simulink model "CryoDetFP"  (R2015b)
settings: Solver=ode45  SolverMode=SingleTasking  StartTime=0.0  StopTime=10e-5  MaxStep=1e-9  RelTol=1e-3
values from neighbouring files (symbols this model uses):
  Fclk = Fadc/2    (= 185000000)    [setupCryoFPGA.m]    (also in setupCryoNew.m)
  freqBusAddrBits = 4    [setupCryoNew.m]
  noise = ifft(exp(2i*pi*rand(1, noiseLen)) .* fft(fir1(noiseLen-1, noiseBW/Fclk*noiseSteps)))    [setupCryoFPGA.m]    (also in setupCryoNew.m = exp(2i*pi*rand(1, noiseLen)))
  noiseLen = 128    [setupCryoFPGA.m]    (also in setupCryoNew.m)
  noiseSteps = 32    [setupCryoFPGA.m]    (also in setupCryoNew.m)
  notch = tf( [1 a*wNotch/Q wNotch^2], [1 wNotch/Q wNotch^2])    [setupCryoNew.m]
  notch2 = tf( [1 a*wNotch/Q wNotch^2], [1 wNotch/Q wNotch^2])    [setupCryoNew.m]
  Tclk = 1/Fclk    (= 5.40540540541e-09)    [setupCryoFPGA.m]    (also in setupCryoNew.m)
undefined symbols (not defined in the file or in its folder): AXI4, Lite, notch3, notch4, xlipgetpartsetting
libraries: xbsIndex_r4 x1085
(part 1 of 8)
settings Model: Creator=ssmith  LastModifiedBy=ssmith
settings DataIOCC: SaveFormat=Array
settings OptimizationCC: BlockReduction=off  BooleanDataType=off
settings DebuggingCC: SaveWithParameterizedLinksMsg=none  UnderspecifiedInitializationDetection=Classic  MergeDetectMultiDrivingBlocksExec=none  SignalResolutionControl=TryResolveAllWithWarning
settings HardwareCC: ProdBitPerPointer=32  ProdLargestAtomicFloat=None  ProdIntDivRoundTo=Undefined  ProdEndianess=Unspecified  ProdWordSize=32  ProdHWDeviceType=32-bit Generic  TargetUnknown=on
settings GRTTargetCC: GeneratePreprocessorConditionals=Disable all
settings ConfigComp: CovModelRefEnable=Off  CovSFcnEnable=off

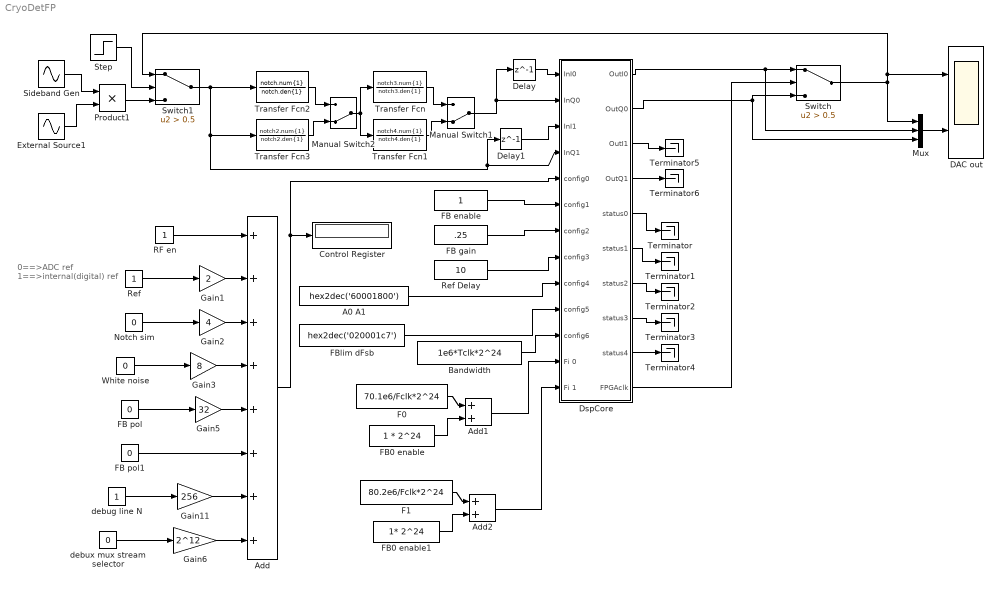
== system CryoDetFP ==
  note: 0==>ADC ref
      | 1==>internal(digital) ref
  A0 A1 : Constant  Value=hex2dec('60001800')  SampleTime=Tclk
  Add : Sum  Inputs=++++++++
  Add1 : Sum
  Add2 : Sum
  Bandwidth : Constant  Value=1e6*Tclk*2^24  SampleTime=Tclk
  Control Register : Display
      settings: Format=hex (Stored Integer)  Decimation=1000
  DAC out : Scope  NumInputPorts=2
  Delay : Delay  DelayLength=1  SampleTime=Tclk/2
  Delay1 : Delay  DelayLength=1  SampleTime=Tclk/2
  DspCore : Subsystem
  External Source1 : Sin  Amplitude=.8  Frequency=2*pi*70.1e6  SampleTime=0
  F0 : Constant  Value=70.1e6/Fclk*2^24  SampleTime=Tclk
  F1 : Constant  Value=80.2e6/Fclk*2^24  SampleTime=Tclk
  FB enable : Constant  SampleTime=Tclk
  FB gain : Constant  Value=.25  SampleTime=Tclk
  FB pol : Constant  Value=0  SampleTime=Tclk
  FB pol1 : Constant  Value=0  SampleTime=Tclk
  FB0 enable : Constant  Value=1 * 2^24  SampleTime=Tclk
  FB0 enable1 : Constant  Value=1* 2^24  SampleTime=Tclk
  FBlim dFsb : Constant  Value=hex2dec('020001c7')  SampleTime=Tclk
  Gain1 : Gain  Gain=2
  Gain11 : Gain  Gain=256
  Gain2 : Gain  Gain=4
  Gain3 : Gain  Gain=8
  Gain5 : Gain  Gain=32
  Gain6 : Gain  Gain=2^12
  Manual Switch1 : ManualSwitch  CurrentSetting=0
  Manual Switch2 : ManualSwitch  CurrentSetting=0
  Mux : Mux  Inputs=3
  Notch sim : Constant  Value=0  SampleTime=Tclk
  Product1 : Product
  RF en : Constant  SampleTime=Tclk
  Ref : Constant  SampleTime=Tclk
  Ref Delay : Constant  Value=10  SampleTime=Tclk
  Sideband Gen : Sin  Amplitude=0.24  Bias=0.75  Frequency=2*pi*1.284e6  SampleTime=0
  Step : Step  Time=1e-5  SampleTime=0
  Switch : Switch  Criteria=u2 > Threshold  Threshold=0.5
  Switch1 : Switch  Criteria=u2 > Threshold  Threshold=0.5
  Terminator{,1..6} (7 alike) : Terminator
  Transfer Fcn : TransferFcn  Numerator=notch3.num{1}  Denominator=notch3.den{1}
  Transfer Fcn1 : TransferFcn  Numerator=notch4.num{1}  Denominator=notch4.den{1}
  Transfer Fcn2 : TransferFcn  Numerator=notch.num{1}  Denominator=notch.den{1}
  Transfer Fcn3 : TransferFcn  Numerator=notch2.num{1}  Denominator=notch2.den{1}
  White noise : Constant  Value=0  SampleTime=Tclk
  debug line N : Constant  SampleTime=Tclk
  debux mux stream selector : Constant  Value=0  SampleTime=Tclk
  wires:
  Add/1 -> DspCore/5(config0), Control Register/1
  FB enable/1 -> DspCore/6(config1)
  DspCore/5(status0) -> Terminator/1
  DspCore/6(status1) -> Terminator1/1
  DspCore/7(status2) -> Terminator2/1
  DspCore/8(status3) -> Terminator3/1
  DspCore/9(status4) -> Terminator4/1
  Sideband Gen/1 -> Product1/1
  DspCore/10(FPGAclk) -> Switch/2
  DspCore/2(OutQ0) -> Switch/3, Mux/3
  Switch/1 -> DAC out/1, Switch1/1, Mux/1
  DspCore/1(OutI0) -> Switch/1, Mux/2
  Product1/1 -> Switch1/3
  Step/1 -> Switch1/2
  Manual Switch1/1 -> Delay/1, DspCore/2(InQ0)
  External Source1/1 -> Product1/2
  Transfer Fcn1/1 -> Manual Switch1/2
  Transfer Fcn/1 -> Manual Switch1/1
  RF en/1 -> Add/1
  Ref/1 -> Gain1/1
  Notch sim/1 -> Gain2/1
  White noise/1 -> Gain3/1
  FB pol/1 -> Gain5/1
  debux mux stream selector/1 -> Gain6/1
  Gain1/1 -> Add/2
  Gain2/1 -> Add/3
  Gain3/1 -> Add/4
  debug line N/1 -> Gain11/1
  Mux/1 -> DAC out/2
  Delay/1 -> DspCore/1(InI0)
  Delay1/1 -> DspCore/3(InI1)
  Gain11/1 -> Add/7
  Gain6/1 -> Add/8
  Gain5/1 -> Add/5
  FB gain/1 -> DspCore/7(config2)
  Ref Delay/1 -> DspCore/8(config3)
  A0 A1/1 -> DspCore/9("config4 ")
  FBlim dFsb/1 -> DspCore/10(config5)
  Bandwidth/1 -> DspCore/11(config6)
  FB pol1/1 -> Add/6
  FB0 enable/1 -> Add1/2
  F0/1 -> Add1/1
  Add1/1 -> DspCore/12(Fi 0)
  DspCore/3(OutI1) -> Terminator5/1
  DspCore/4(OutQ1) -> Terminator6/1
  Transfer Fcn3/1 -> Manual Switch2/2
  Transfer Fcn2/1 -> Manual Switch2/1
  Switch1/1 -> Transfer Fcn2/1, Transfer Fcn3/1, Delay1/1, DspCore/4(InQ1)
  Manual Switch2/1 -> Transfer Fcn/1, Transfer Fcn1/1
  FB0 enable1/1 -> Add2/2
  F1/1 -> Add2/1
  Add2/1 -> DspCore/13(Fi 1)

== system CryoDetFP/DspCore ==
  note: create an edge to synchronize external DAC interleaver simulation in Simulink
  note: DAC outputs
      | 16 bits
  note: ADC Inputs
      | 16 bits
      | 370 MSPS
  note: FPGA reset
  InI0 : Inport
  InQ0 : Inport  Port=2
  InI1 : Inport  Port=3
  InQ1 : Inport  Port=4
  config0 : Inport  Port=5
  config1 : Inport  Port=6
  config2 : Inport  Port=7
  config3 : Inport  Port=8
  "config4 " : Inport  Port=9
  config5 : Inport  Port=10
  config6 : Inport  Port=11
  Fi 0 : Inport  Port=12
  Fi 1 : Inport  Port=13
  " System Generator1" : xbsIndex_r4/ System Generator  Tag=genX  xilinxfamily=kintexu  part=xcku040  speed=-2-e  package=ffva1156  synthesis_tool=Vivado  clock_wrapper=Clock Enables  directory=./netlist  proj_type=Vivado  Synth_file=Vivado Synthesis Defaults  Impl_file=Vivado Implementation Defaults  testbench=off  simulink_period=Tclk  sysclk_period=Tclk*1e9  dcm_input_clock_period=10  incr_netlist=off  trim_vbits=Everywhere in SubSystem  dbl_ovrd=According to Block Masks  core_generation=According to Block Masks  run_coregen=off  deprecated_control=off  eval_field=0  block_type=sysgen
  AdcDac 0 : Subsystem
  AdcDac 1 : Subsystem
  Configuration : Subsystem
  Constant1 : Constant  Value=0
  Constant2 : Constant  Value=0
  DAC demux clock : Subsystem
  Demux : Demux  Outputs=2
  Demux1 : Demux  Outputs=2
  Mux : Mux  Inputs=2
  Mux1 : Mux  Inputs=2
  Register : xbsIndex_r4/Register  init=1  rst=off  en=off  dbl_ovrd=off  block_type=register
  Step : Step  Time=3e-7  Before=1  After=0  SampleTime=0
  Terminator{1..2,4..9} (8 alike) : Terminator
  fromdsp_dacdata0_0 : xbsIndex_r4/Gateway Out  inherit_from_input=on  hdl_port=on  rows=1  columns=1  UseAsDAC=off  DACChannel='1'  interface=None  automatic_assignment=on  address_offset=hex2dec('00')  intf_name=''  intf_description=''  timing_constraint=None  locs_specified=off  LOCs={}  io_standard={}  block_type=gatewayout
  fromdsp_dacdata0_1 : xbsIndex_r4/Gateway Out  inherit_from_input=on  hdl_port=on  rows=1  columns=1  UseAsDAC=off  DACChannel='1'  interface=None  automatic_assignment=on  address_offset=hex2dec('00')  intf_name=''  intf_description=''  timing_constraint=None  locs_specified=off  LOCs={}  io_standard={}  block_type=gatewayout
  fromdsp_dacdata1_0 : xbsIndex_r4/Gateway Out  inherit_from_input=on  hdl_port=on  rows=1  columns=1  UseAsDAC=off  DACChannel='1'  interface=None  automatic_assignment=on  address_offset=hex2dec('00')  intf_name=''  intf_description=''  timing_constraint=None  locs_specified=off  LOCs={}  io_standard={}  block_type=gatewayout
  fromdsp_dacdata1_1 : xbsIndex_r4/Gateway Out  inherit_from_input=off  hdl_port=on  rows=1  columns=1  UseAsDAC=off  DACChannel='1'  interface=None  automatic_assignment=on  address_offset=hex2dec('00')  intf_name=''  intf_description=''  timing_constraint=None  locs_specified=off  LOCs={}  io_standard={}  block_type=gatewayout
  rst : xbsIndex_r4/Gateway In  gui_display_data_type=Boolean  arith_type=Boolean  n_bits=16  bin_pt=14  preci_type=Single  exp_width=8  frac_width=24  rows=1  columns=1  quantization="Round  (unbiased: +/- Inf)"  overflow=Saturate  period=Tclk  UseAsADC=off  ADCChannel='1'  interface=None  automatic_assignment=on  address_offset=hex2dec('00')  intf_name=''  intf_description=''  timing_constraint=None  locs_specified=off  LOCs={}  io_standard={}  inherit_from_input=off  hdl_port=on  dbl_ovrd=off  block_type=gatewayin
  todsp_adcdata0_0 : xbsIndex_r4/Gateway In  gui_display_data_type=Fixed-point  arith_type="Signed  (2's comp)"  n_bits=16  bin_pt=15  preci_type=Single  exp_width=8  frac_width=24  rows=1  columns=1  quantization=Truncate  overflow=Wrap  period=Tclk  UseAsADC=off  ADCChannel='1'  interface=None  automatic_assignment=on  address_offset=hex2dec('00')  intf_name=''  intf_description=''  timing_constraint=None  locs_specified=off  LOCs={}  io_standard={}  inherit_from_input=off  hdl_port=on  dbl_ovrd=off  block_type=gatewayin
  todsp_adcdata0_1 : xbsIndex_r4/Gateway In  gui_display_data_type=Fixed-point  arith_type="Signed  (2's comp)"  n_bits=16  bin_pt=15  preci_type=Single  exp_width=8  frac_width=24  rows=1  columns=1  quantization=Truncate  overflow=Wrap  period=Tclk  UseAsADC=off  ADCChannel='1'  interface=None  automatic_assignment=on  address_offset=hex2dec('00')  intf_name=''  intf_description=''  timing_constraint=None  locs_specified=off  LOCs={}  io_standard={}  inherit_from_input=off  hdl_port=on  dbl_ovrd=off  block_type=gatewayin
  todsp_adcdata1_0 : xbsIndex_r4/Gateway In  gui_display_data_type=Fixed-point  arith_type="Signed  (2's comp)"  n_bits=16  bin_pt=15  preci_type=Single  exp_width=8  frac_width=24  rows=1  columns=1  quantization=Truncate  overflow=Wrap  period=Tclk  UseAsADC=off  ADCChannel='1'  interface=None  automatic_assignment=on  address_offset=hex2dec('00')  intf_name=''  intf_description=''  timing_constraint=None  locs_specified=off  LOCs={}  io_standard={}  inherit_from_input=off  hdl_port=on  dbl_ovrd=off  block_type=gatewayin
  todsp_adcdata1_1 : xbsIndex_r4/Gateway In  gui_display_data_type=Fixed-point  arith_type="Signed  (2's comp)"  n_bits=16  bin_pt=15  preci_type=Single  exp_width=8  frac_width=24  rows=1  columns=1  quantization=Truncate  overflow=Wrap  period=Tclk  UseAsADC=off  ADCChannel='1'  interface=None  automatic_assignment=on  address_offset=hex2dec('00')  intf_name=''  intf_description=''  timing_constraint=None  locs_specified=off  LOCs={}  io_standard={}  inherit_from_input=off  hdl_port=on  dbl_ovrd=off  block_type=gatewayin
  todsp_adcdata2_0 : xbsIndex_r4/Gateway In  gui_display_data_type=Fixed-point  arith_type="Signed  (2's comp)"  n_bits=16  bin_pt=15  preci_type=Single  exp_width=8  frac_width=24  rows=1  columns=1  quantization=Truncate  overflow=Wrap  period=Tclk  UseAsADC=off  ADCChannel='1'  interface=None  automatic_assignment=on  address_offset=hex2dec('00')  intf_name=''  intf_description=''  timing_constraint=None  locs_specified=off  LOCs={}  io_standard={}  inherit_from_input=off  hdl_port=on  dbl_ovrd=off  block_type=gatewayin
  todsp_adcdata2_1 : xbsIndex_r4/Gateway In  gui_display_data_type=Fixed-point  arith_type="Signed  (2's comp)"  n_bits=16  bin_pt=15  preci_type=Single  exp_width=8  frac_width=24  rows=1  columns=1  quantization=Truncate  overflow=Wrap  period=Tclk  UseAsADC=off  ADCChannel='1'  interface=None  automatic_assignment=on  address_offset=hex2dec('00')  intf_name=''  intf_description=''  timing_constraint=None  locs_specified=off  LOCs={}  io_standard={}  inherit_from_input=off  hdl_port=on  dbl_ovrd=off  block_type=gatewayin
  todsp_adcdata3_0 : xbsIndex_r4/Gateway In  gui_display_data_type=Fixed-point  arith_type="Signed  (2's comp)"  n_bits=16  bin_pt=15  preci_type=Single  exp_width=8  frac_width=24  rows=1  columns=1  quantization=Truncate  overflow=Wrap  period=Tclk  UseAsADC=off  ADCChannel='1'  interface=None  automatic_assignment=on  address_offset=hex2dec('00')  intf_name=''  intf_description=''  timing_constraint=None  locs_specified=off  LOCs={}  io_standard={}  inherit_from_input=off  hdl_port=on  dbl_ovrd=off  block_type=gatewayin
  todsp_adcdata3_1 : xbsIndex_r4/Gateway In  gui_display_data_type=Fixed-point  arith_type="Signed  (2's comp)"  n_bits=16  bin_pt=15  preci_type=Single  exp_width=8  frac_width=24  rows=1  columns=1  quantization=Truncate  overflow=Wrap  period=Tclk  UseAsADC=off  ADCChannel='1'  interface=None  automatic_assignment=on  address_offset=hex2dec('00')  intf_name=''  intf_description=''  timing_constraint=None  locs_specified=off  LOCs={}  io_standard={}  inherit_from_input=off  hdl_port=on  dbl_ovrd=off  block_type=gatewayin
  todsp_adcdata4_0 : xbsIndex_r4/Gateway In  gui_display_data_type=Fixed-point  arith_type="Signed  (2's comp)"  n_bits=16  bin_pt=15  preci_type=Single  exp_width=8  frac_width=24  rows=1  columns=1  quantization=Truncate  overflow=Wrap  period=Tclk  UseAsADC=off  ADCChannel='1'  interface=None  automatic_assignment=on  address_offset=hex2dec('00')  intf_name=''  intf_description=''  timing_constraint=None  locs_specified=off  LOCs={}  io_standard={}  inherit_from_input=off  hdl_port=on  dbl_ovrd=off  block_type=gatewayin
  todsp_adcdata4_1 : xbsIndex_r4/Gateway In  gui_display_data_type=Fixed-point  arith_type="Signed  (2's comp)"  n_bits=16  bin_pt=15  preci_type=Single  exp_width=8  frac_width=24  rows=1  columns=1  quantization=Truncate  overflow=Wrap  period=Tclk  UseAsADC=off  ADCChannel='1'  interface=None  automatic_assignment=on  address_offset=hex2dec('00')  intf_name=''  intf_description=''  timing_constraint=None  locs_specified=off  LOCs={}  io_standard={}  inherit_from_input=off  hdl_port=on  dbl_ovrd=off  block_type=gatewayin
  todsp_adcdata5_0 : xbsIndex_r4/Gateway In  gui_display_data_type=Fixed-point  arith_type="Signed  (2's comp)"  n_bits=16  bin_pt=15  preci_type=Single  exp_width=8  frac_width=24  rows=1  columns=1  quantization=Truncate  overflow=Wrap  period=Tclk  UseAsADC=off  ADCChannel='1'  interface=None  automatic_assignment=on  address_offset=hex2dec('00')  intf_name=''  intf_description=''  timing_constraint=None  locs_specified=off  LOCs={}  io_standard={}  inherit_from_input=off  hdl_port=on  dbl_ovrd=off  block_type=gatewayin
  todsp_adcdata5_1 : xbsIndex_r4/Gateway In  gui_display_data_type=Fixed-point  arith_type="Signed  (2's comp)"  n_bits=16  bin_pt=15  preci_type=Single  exp_width=8  frac_width=24  rows=1  columns=1  quantization=Truncate  overflow=Wrap  period=Tclk  UseAsADC=off  ADCChannel='1'  interface=None  automatic_assignment=on  address_offset=hex2dec('00')  intf_name=''  intf_description=''  timing_constraint=None  locs_specified=off  LOCs={}  io_standard={}  inherit_from_input=off  hdl_port=on  dbl_ovrd=off  block_type=gatewayin
  OutI0 : Outport
  OutQ0 : Outport  Port=2
  OutI1 : Outport  Port=3
  OutQ1 : Outport  Port=4
  status0 : Outport  Port=5
  status1 : Outport  Port=6
  status2 : Outport  Port=7
  status3 : Outport  Port=8
  status4 : Outport  Port=9
  FPGAclk : Outport  Port=10
  tag scope: fpgaReset=global
  wires:
  InI0/1 -> todsp_adcdata0_0/1
  fromdsp_dacdata1_0/1 -> OutI1/1
  fromdsp_dacdata0_0/1 -> OutI0/1
  InI1/1 -> todsp_adcdata1_0/1
  Step/1 -> rst/1
  rst/1 -> Register/1
  todsp_adcdata2_0/1 -> Terminator1/1
  todsp_adcdata3_0/1 -> Terminator2/1
  todsp_adcdata4_0/1 -> Terminator4/1
  todsp_adcdata5_0/1 -> Terminator5/1
  InQ0/1 -> todsp_adcdata0_1/1
  fromdsp_dacdata0_1/1 -> OutQ0/1
  fromdsp_dacdata1_1/1 -> OutQ1/1
  InQ1/1 -> todsp_adcdata1_1/1
  todsp_adcdata2_1/1 -> Terminator6/1
  todsp_adcdata3_1/1 -> Terminator7/1
  todsp_adcdata4_1/1 -> Terminator8/1
  todsp_adcdata5_1/1 -> Terminator9/1
  Configuration/1(Out1) -> status0/1
  Configuration/2(Out2) -> status1/1
  Configuration/3(Out3) -> status2/1
  Configuration/4(Out4) -> status3/1
  Configuration/5(Out5) -> status4/1
  Constant1/1 -> todsp_adcdata3_0/1, todsp_adcdata3_1/1, todsp_adcdata4_1/1, todsp_adcdata5_0/1, todsp_adcdata5_1/1, todsp_adcdata4_0/1, todsp_adcdata2_1/1, todsp_adcdata2_0/1
  DAC demux clock/1(IQtoggle) -> FPGAclk/1
  Demux/2 -> fromdsp_dacdata0_1/1
  Demux/1 -> fromdsp_dacdata0_0/1
  Mux/1 -> AdcDac 0/1(ADCin)
  AdcDac 0/1(DACout) -> Demux/1
  todsp_adcdata0_0/1 -> Mux/1
  todsp_adcdata0_1/1 -> Mux/2
  Demux1/2 -> DAC demux clock/1(In1), fromdsp_dacdata1_1/1
  Mux1/1 -> AdcDac 1/1(In1)
  AdcDac 1/1(Out1) -> Demux1/1
  todsp_adcdata1_0/1 -> Mux1/1
  todsp_adcdata1_1/1 -> Mux1/2
  Demux1/1 -> fromdsp_dacdata1_0/1
  config0/1 -> Configuration/2(config0)
  config1/1 -> Configuration/3(config1)
  config2/1 -> Configuration/4(config2)
  config3/1 -> Configuration/5(config3)
  "config4 "/1 -> Configuration/6(config4)
  config5/1 -> Configuration/7(config5)
  config6/1 -> Configuration/8(config6)
  Fi 0/1 -> Configuration/9("Fi 0 ")
  Register/1 -> [fpgaReset]
  Constant2/1 -> Configuration/20(Fi 11), Configuration/19(Fi 10), Configuration/18(Fi 9), Configuration/17(Fi 8), Configuration/16(Fi 7), Configuration/15(Fi 6), Configuration/14(Fi 5), Configuration/13(Fi 4), Configuration/12(Fi 3), Configuration/11(Fi 2), Configuration/1(config63), Configuration/21(In13)
  Fi 1/1 -> Configuration/10(Fi 1)

== system CryoDetFP/DspCore/AdcDac 0 ==
  note: reference
  ADCin : Inport
  Goto Tag Visibility : GotoTagVisibility  GotoTag=freqBus
  Goto Tag Visibility1 : GotoTagVisibility  GotoTag=dphiBus
  Goto Tag Visibility2 : GotoTagVisibility  GotoTag=dFbus
  Mux : Mux  Inputs=2
  Ref Delay : Subsystem
  SBmodulator : Subsystem
  Terminator : Terminator
  dF : Subsystem
  dphi : Subsystem
  eta : Subsystem
  loopFilter : Subsystem
  twelveLineUDC 0 : Subsystem
  twelveLineUDC 1 : Subsystem
  DACout : Outport
  wires:
  twelveLineUDC 1/1(Out1) -> Terminator/1
  twelveLineUDC 0/1(toDAC) -> SBmodulator/1(In1)
  ADCin/1 -> Mux/1
  Ref Delay/1(Out1) -> Mux/2
  Mux/1 -> twelveLineUDC 1/1(In1), twelveLineUDC 0/1(In1)
  twelveLineUDC 0/2(demodulated) -> dF/1(In1), eta/1(In1)
  dF/1(Out1) -> loopFilter/1(In1)
  SBmodulator/1(Out1) -> Ref Delay/1(In1), DACout/1
  eta/1(etaBus) -> dF/2(etaBus)
  loopFilter/1(Out1) -> dphi/1(In1)

== system CryoDetFP/DspCore/AdcDac 1 ==
  note: AdcDac1
      | eventually is a copy of AdcDac0
      | to handle 2nd ADC-DAC pair
      | dummy for now
      | it must output DAC values for 2nd DAC
  In1 : Inport
  Constant : xbsIndex_r4/Constant  const=0  gui_display_data_type=Fixed-point  arith_type=Signed (2's comp)  n_bits=16  bin_pt=14  preci_type=Single  exp_width=8  frac_width=24  explicit_period=on  period=Tclk  equ=P=C  opselect=C  inp2=PCIN>>17  opr=+  inp1=P  carry=CIN  dbl_ovrd=off  block_type=constant
  Mux : Mux  Inputs=2
  Terminator : Terminator
  Out1 : Outport
  wires:
  Constant/1 -> Mux/2, Mux/1
  Mux/1 -> Out1/1
  In1/1 -> Terminator/1

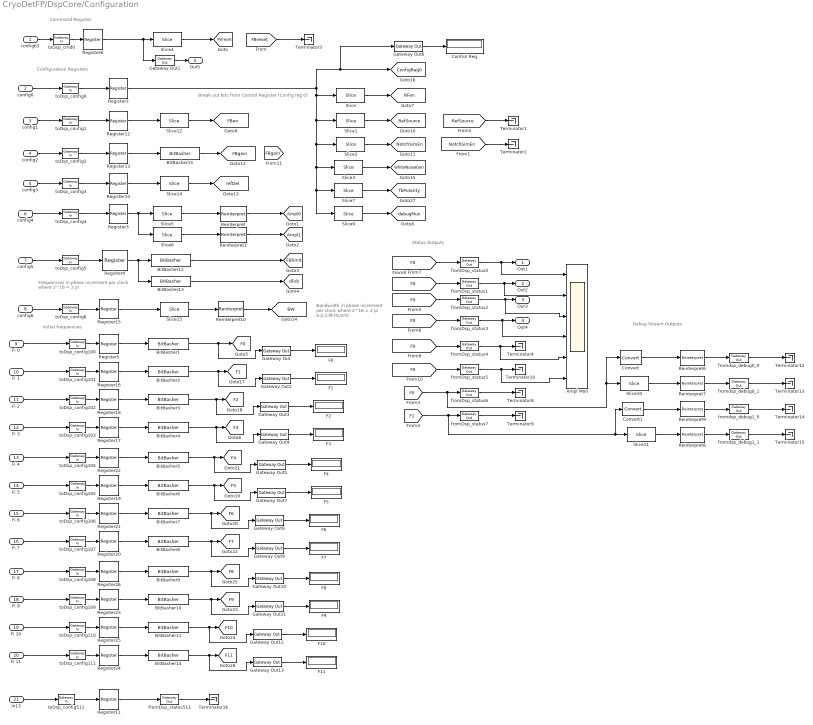
== system CryoDetFP/DspCore/Configuration ==
  note: Status Outputs
  note: Frequencies in phase increment per clock
      | where 2^16 = 2 pi
  note: initial frequencies
  note: Configuration Registers
  note: Command Register
  note: Break out bits from Control Register (Config reg 0)
  note: Debug Stream Outputs
  note: Bandwidth in phase increment per clock
      | where 2^16 = 2 pi e.g 2.8kHz/unit
  config63 : Inport
  config0 : Inport  Port=2
  config1 : Inport  Port=3
  config2 : Inport  Port=4
  config3 : Inport  Port=5
  config4 : Inport  Port=6
  config5 : Inport  Port=7
  config6 : Inport  Port=8
  "Fi 0 " : Inport  Port=9
  Fi 1 : Inport  Port=10
  Fi 2 : Inport  Port=11
  Fi 3 : Inport  Port=12
  Fi 4 : Inport  Port=13
  Fi 5 : Inport  Port=14
  Fi 6 : Inport  Port=15
  Fi 7 : Inport  Port=16
  Fi 8 : Inport  Port=17
  Fi 9 : Inport  Port=18
  Fi 10 : Inport  Port=19
  Fi 11 : Inport  Port=20
  In13 : Inport  Port=21
  Ampl Mon : Scope  NumInputPorts=6
  BitBasher{1..11,14} (12 alike) : xbsIndex_r4/BitBasher  bitexpr=a={b[24:0]}  display_expr=on  sr_1=a  arith_type1=Unsigned  bin_pt1=0  sr_2=2  arith_type2=Unsigned  bin_pt2=0  sr_3=3  arith_type3=Unsigned  bin_pt3=0  sr_4=4  arith_type4=Unsigned  bin_pt4=0  dbl_ovrd=off  block_type=bitbasher
  BitBasher12 : xbsIndex_r4/BitBasher  bitexpr=a={b[31:16]}  display_expr=on  sr_1=a  arith_type1=Unsigned  bin_pt1=16  sr_2=2  arith_type2=Unsigned  bin_pt2=0  sr_3=3  arith_type3=Unsigned  bin_pt3=0  sr_4=4  arith_type4=Unsigned  bin_pt4=0  dbl_ovrd=off  block_type=bitbasher
  BitBasher13 : xbsIndex_r4/BitBasher  bitexpr=a={b[15:0]}  display_expr=on  sr_1=a  arith_type1=Unsigned  bin_pt1=16  sr_2=2  arith_type2=Unsigned  bin_pt2=0  sr_3=3  arith_type3=Unsigned  bin_pt3=0  sr_4=4  arith_type4=Unsigned  bin_pt4=0  dbl_ovrd=off  block_type=bitbasher
  BitBasher15 : xbsIndex_r4/BitBasher  bitexpr=a={b[15:0]}  display_expr=on  sr_1=a  arith_type1=Unsigned  bin_pt1=12  sr_2=2  arith_type2=Unsigned  bin_pt2=0  sr_3=3  arith_type3=Unsigned  bin_pt3=0  sr_4=4  arith_type4=Unsigned  bin_pt4=0  dbl_ovrd=off  block_type=bitbasher
  Control Reg : Display
  Convert : xbsIndex_r4/Convert  gui_display_data_type=Fixed-point  arith_type="Signed  (2's comp)"  n_bits=16  bin_pt=7  float_type=Single  exp_bits=8  fraction_bits=24  quantization=Truncate  overflow=Wrap  en=off  latency=0  pipeline=off  dbl_ovrd=off  block_type=convert
  Convert1 : xbsIndex_r4/Convert  gui_display_data_type=Fixed-point  arith_type="Signed  (2's comp)"  n_bits=16  bin_pt=7  float_type=Single  exp_bits=8  fraction_bits=24  quantization=Truncate  overflow=Wrap  en=off  latency=0  pipeline=off  dbl_ovrd=off  block_type=convert
  F{0..11} (12 alike) : Display
  Gateway Out{,2..5,7..13} (12 alike) : xbsIndex_r4/Gateway Out  inherit_from_input=on  hdl_port=off  rows=1  columns=1  UseAsDAC=off  DACChannel='1'  interface=None  automatic_assignment=on  address_offset=hex2dec('00')  intf_name=''  intf_description=''  timing_constraint=None  locs_specified=off  LOCs={}  io_standard={}  block_type=gatewayout
  Gateway Out1 : xbsIndex_r4/Gateway Out  inherit_from_input=off  hdl_port=off  rows=1  columns=1  UseAsDAC=off  DACChannel='1'  interface=None  automatic_assignment=on  address_offset=hex2dec('00')  intf_name=''  intf_description=''  timing_constraint=None  locs_specified=off  LOCs={}  io_standard={}  block_type=gatewayout
  Gateway Out6 : xbsIndex_r4/Gateway Out  inherit_from_input=off  hdl_port=off  rows=1  columns=1  UseAsDAC=off  DACChannel='1'  interface=None  automatic_assignment=on  address_offset=hex2dec('00')  intf_name=''  intf_description=''  timing_constraint=None  locs_specified=off  LOCs={}  io_standard={}  block_type=gatewayout
  Register{2..6,11..26} (21 alike) : xbsIndex_r4/Register  init=0  rst=off  en=off  dbl_ovrd=off  block_type=register
  Reinterpret : xbsIndex_r4/Reinterpret  force_arith_type=on  arith_type=Unsigned  force_bin_pt=on  bin_pt=16  block_type=reinterpret
  Reinterpret1 : xbsIndex_r4/Reinterpret  force_arith_type=on  arith_type=Unsigned  force_bin_pt=on  bin_pt=16  block_type=reinterpret
  Reinterpret10 : xbsIndex_r4/Reinterpret  force_arith_type=on  arith_type=Unsigned  force_bin_pt=on  bin_pt=16  block_type=reinterpret
  Reinterpret{6..9} (4 alike) : xbsIndex_r4/Reinterpret  force_arith_type=on  arith_type="Signed  (2's comp)"  force_bin_pt=on  bin_pt=15  block_type=reinterpret
  Slice : xbsIndex_r4/Slice  nbits=1  boolean_output=on  mode=Upper Bit Location + Width  bit1=0  base1=LSB of Input  bit0=0  base0=LSB of Input  dbl_ovrd=off  block_type=slice
  Slice1 : xbsIndex_r4/Slice  nbits=1  boolean_output=on  mode=Upper Bit Location + Width  bit1=1  base1=LSB of Input  bit0=0  base0=LSB of Input  dbl_ovrd=off  block_type=slice
  Slice10 : xbsIndex_r4/Slice  nbits=16  boolean_output=off  mode=Lower Bit Location + Width  bit1=0  base1=MSB of Input  bit0=0  base0=LSB of Input  dbl_ovrd=off  block_type=slice
  Slice11 : xbsIndex_r4/Slice  nbits=16  boolean_output=off  mode=Lower Bit Location + Width  bit1=0  base1=MSB of Input  bit0=0  base0=LSB of Input  dbl_ovrd=off  block_type=slice
  Slice12 : xbsIndex_r4/Slice  nbits=1  boolean_output=on  mode=Upper Bit Location + Width  bit1=0  base1=LSB of Input  bit0=0  base0=LSB of Input  dbl_ovrd=off  block_type=slice
  Slice14 : xbsIndex_r4/Slice  nbits=8  boolean_output=off  mode=Lower Bit Location + Width  bit1=0  base1=LSB of Input  bit0=0  base0=LSB of Input  dbl_ovrd=off  block_type=slice
  Slice15 : xbsIndex_r4/Slice  nbits=16  boolean_output=off  mode=Lower Bit Location + Width  bit1=0  base1=LSB of Input  bit0=0  base0=LSB of Input  dbl_ovrd=off  block_type=slice
  Slice2 : xbsIndex_r4/Slice  nbits=1  boolean_output=on  mode=Upper Bit Location + Width  bit1=2  base1=LSB of Input  bit0=0  base0=LSB of Input  dbl_ovrd=off  block_type=slice
  Slice3 : xbsIndex_r4/Slice  nbits=1  boolean_output=on  mode=Upper Bit Location + Width  bit1=3  base1=LSB of Input  bit0=0  base0=LSB of Input  dbl_ovrd=off  block_type=slice
  Slice4 : xbsIndex_r4/Slice  nbits=1  boolean_output=on  mode=Upper Bit Location + Width  bit1=0  base1=LSB of Input  bit0=0  base0=LSB of Input  dbl_ovrd=off  block_type=slice
  Slice5 : xbsIndex_r4/Slice  nbits=16  boolean_output=off  mode=Upper Bit Location + Width  bit1=31  base1=LSB of Input  bit0=0  base0=LSB of Input  dbl_ovrd=off  block_type=slice
  Slice6 : xbsIndex_r4/Slice  nbits=16  boolean_output=off  mode=Upper Bit Location + Width  bit1=15  base1=LSB of Input  bit0=0  base0=LSB of Input  dbl_ovrd=off  block_type=slice
  Slice7 : xbsIndex_r4/Slice  nbits=1  boolean_output=on  mode=Upper Bit Location + Width  bit1=4  base1=LSB of Input  bit0=0  base0=LSB of Input  dbl_ovrd=off  block_type=slice
  Slice9 : xbsIndex_r4/Slice  nbits=8  boolean_output=off  mode=Lower Bit Location + Width  bit1=6  base1=LSB of Input  bit0=8  base0=LSB of Input  dbl_ovrd=off  block_type=slice
  Terminator{1..4,8..10,12..16} (12 alike) : Terminator
  fromDsp_status0 : xbsIndex_r4/Gateway Out  inherit_from_input=on  hdl_port=on  rows=1  columns=1  UseAsDAC=off  DACChannel='1'  interface=AXI4-Lite  automatic_assignment=off  address_offset=hex2dec('00')  intf_name=''  intf_description=''  timing_constraint=None  locs_specified=off  LOCs={}  io_standard={}  block_type=gatewayout
  fromDsp_status1 : xbsIndex_r4/Gateway Out  inherit_from_input=on  hdl_port=on  rows=1  columns=1  UseAsDAC=off  DACChannel='1'  interface=AXI4-Lite  automatic_assignment=off  address_offset=hex2dec('04')  intf_name=''  intf_description=''  timing_constraint=None  locs_specified=off  LOCs={}  io_standard={}  block_type=gatewayout
  fromDsp_status2 : xbsIndex_r4/Gateway Out  inherit_from_input=on  hdl_port=on  rows=1  columns=1  UseAsDAC=off  DACChannel='1'  interface=AXI4-Lite  automatic_assignment=off  address_offset=hex2dec('08')  intf_name=''  intf_description=''  timing_constraint=None  locs_specified=off  LOCs={}  io_standard={}  block_type=gatewayout
  fromDsp_status3 : xbsIndex_r4/Gateway Out  inherit_from_input=on  hdl_port=on  rows=1  columns=1  UseAsDAC=off  DACChannel='1'  interface=AXI4-Lite  automatic_assignment=off  address_offset=hex2dec('0C')  intf_name=''  intf_description=''  timing_constraint=None  locs_specified=off  LOCs={}  io_standard={}  block_type=gatewayout
  fromDsp_status4 : xbsIndex_r4/Gateway Out  inherit_from_input=on  hdl_port=on  rows=1  columns=1  UseAsDAC=off  DACChannel='1'  interface=AXI4-Lite  automatic_assignment=off  address_offset=hex2dec('10')  intf_name=''  intf_description=''  timing_constraint=None  locs_specified=off  LOCs={}  io_standard={}  block_type=gatewayout
  fromDsp_status5 : xbsIndex_r4/Gateway Out  inherit_from_input=on  hdl_port=on  rows=1  columns=1  UseAsDAC=off  DACChannel='1'  interface=AXI4-Lite  automatic_assignment=off  address_offset=hex2dec('14')  intf_name=''  intf_description=''  timing_constraint=None  locs_specified=off  LOCs={}  io_standard={}  block_type=gatewayout
  fromDsp_status511 : xbsIndex_r4/Gateway Out  inherit_from_input=on  hdl_port=on  rows=1  columns=1  UseAsDAC=off  DACChannel='1'  interface=AXI4-Lite  automatic_assignment=off  address_offset=hex2dec('7FC')  intf_name=''  intf_description=''  timing_constraint=None  locs_specified=off  LOCs={}  io_standard={}  block_type=gatewayout
  fromDsp_status6 : xbsIndex_r4/Gateway Out  inherit_from_input=on  hdl_port=on  rows=1  columns=1  UseAsDAC=off  DACChannel='1'  interface=AXI4-Lite  automatic_assignment=off  address_offset=hex2dec('18')  intf_name=''  intf_description=''  timing_constraint=None  locs_specified=off  LOCs={}  io_standard={}  block_type=gatewayout
  fromDsp_status7 : xbsIndex_r4/Gateway Out  inherit_from_input=on  hdl_port=on  rows=1  columns=1  UseAsDAC=off  DACChannel='1'  interface=AXI4-Lite  automatic_assignment=off  address_offset=hex2dec('1C')  intf_name=''  intf_description=''  timing_constraint=None  locs_specified=off  LOCs={}  io_standard={}  block_type=gatewayout
  fromdsp_debug0_0 : xbsIndex_r4/Gateway Out  inherit_from_input=on  hdl_port=on  rows=1  columns=1  UseAsDAC=off  DACChannel='1'  interface=None  automatic_assignment=on  address_offset=hex2dec('00')  intf_name=''  intf_description=''  timing_constraint=None  locs_specified=off  LOCs={}  io_standard={}  block_type=gatewayout
  fromdsp_debug0_1 : xbsIndex_r4/Gateway Out  inherit_from_input=on  hdl_port=on  rows=1  columns=1  UseAsDAC=off  DACChannel='1'  interface=None  automatic_assignment=on  address_offset=hex2dec('00')  intf_name=''  intf_description=''  timing_constraint=None  locs_specified=off  LOCs={}  io_standard={}  block_type=gatewayout
  fromdsp_debug1_0 : xbsIndex_r4/Gateway Out  inherit_from_input=on  hdl_port=on  rows=1  columns=1  UseAsDAC=off  DACChannel='1'  interface=None  automatic_assignment=on  address_offset=hex2dec('00')  intf_name=''  intf_description=''  timing_constraint=None  locs_specified=off  LOCs={}  io_standard={}  block_type=gatewayout
  fromdsp_debug1_1 : xbsIndex_r4/Gateway Out  inherit_from_input=off  hdl_port=on  rows=1  columns=1  UseAsDAC=off  DACChannel='1'  interface=None  automatic_assignment=on  address_offset=hex2dec('00')  intf_name=''  intf_description=''  timing_constraint=None  locs_specified=off  LOCs={}  io_standard={}  block_type=gatewayout
  toDsp_cmd0 : xbsIndex_r4/Gateway In  gui_display_data_type=Fixed-point  arith_type=Unsigned  n_bits=32  bin_pt=0  preci_type=Single  exp_width=8  frac_width=24  rows=1  columns=1  quantization=Truncate  overflow=Wrap  period=Tclk  UseAsADC=off  ADCChannel='1'  interface=AXI4-Lite  automatic_assignment=off  address_offset=hex2dec('8fc')  intf_name=''  intf_description=''  timing_constraint=None  locs_specified=off  LOCs={}  io_standard={}  inherit_from_input=off  hdl_port=on  dbl_ovrd=off  block_type=gatewayin
  toDsp_config0 : xbsIndex_r4/Gateway In  gui_display_data_type=Fixed-point  arith_type=Unsigned  n_bits=32  bin_pt=0  preci_type=Single  exp_width=8  frac_width=24  rows=1  columns=1  quantization=Truncate  overflow=Wrap  period=Tclk  UseAsADC=off  ADCChannel='1'  interface=AXI4-Lite  automatic_assignment=off  address_offset=hex2dec('800')  intf_name=''  intf_description=''  timing_constraint=None  locs_specified=off  LOCs={}  io_standard={}  inherit_from_input=off  hdl_port=on  dbl_ovrd=off  block_type=gatewayin
  toDsp_config1 : xbsIndex_r4/Gateway In  gui_display_data_type=Fixed-point  arith_type=Unsigned  n_bits=32  bin_pt=0  preci_type=Single  exp_width=8  frac_width=24  rows=1  columns=1  quantization=Truncate  overflow=Wrap  period=Tclk  UseAsADC=off  ADCChannel='1'  interface=AXI4-Lite  automatic_assignment=off  address_offset=hex2dec('804')  intf_name=''  intf_description=''  timing_constraint=None  locs_specified=off  LOCs={}  io_standard={}  inherit_from_input=off  hdl_port=on  dbl_ovrd=off  block_type=gatewayin
  toDsp_config100 : xbsIndex_r4/Gateway In  gui_display_data_type=Fixed-point  arith_type=Unsigned  n_bits=32  bin_pt=0  preci_type=Single  exp_width=8  frac_width=24  rows=1  columns=1  quantization=Truncate  overflow=Wrap  period=Tclk  UseAsADC=off  ADCChannel='1'  interface=AXI4-Lite  automatic_assignment=off  address_offset=hex2dec('900')  intf_name=''  intf_description=''  timing_constraint=None  locs_specified=off  LOCs={}  io_standard={}  inherit_from_input=off  hdl_port=on  dbl_ovrd=off  block_type=gatewayin
  toDsp_config101 : xbsIndex_r4/Gateway In  gui_display_data_type=Fixed-point  arith_type=Unsigned  n_bits=32  bin_pt=0  preci_type=Single  exp_width=8  frac_width=24  rows=1  columns=1  quantization=Truncate  overflow=Wrap  period=Tclk  UseAsADC=off  ADCChannel='1'  interface=AXI4-Lite  automatic_assignment=off  address_offset=hex2dec('904')  intf_name=''  intf_description=''  timing_constraint=None  locs_specified=off  LOCs={}  io_standard={}  inherit_from_input=off  hdl_port=on  dbl_ovrd=off  block_type=gatewayin
  toDsp_config102 : xbsIndex_r4/Gateway In  gui_display_data_type=Fixed-point  arith_type=Unsigned  n_bits=32  bin_pt=0  preci_type=Single  exp_width=8  frac_width=24  rows=1  columns=1  quantization=Truncate  overflow=Wrap  period=Tclk  UseAsADC=off  ADCChannel='1'  interface=AXI4-Lite  automatic_assignment=off  address_offset=hex2dec('908')  intf_name=''  intf_description=''  timing_constraint=None  locs_specified=off  LOCs={}  io_standard={}  inherit_from_input=off  hdl_port=on  dbl_ovrd=off  block_type=gatewayin
  toDsp_config103 : xbsIndex_r4/Gateway In  gui_display_data_type=Fixed-point  arith_type=Unsigned  n_bits=32  bin_pt=0  preci_type=Single  exp_width=8  frac_width=24  rows=1  columns=1  quantization=Truncate  overflow=Wrap  period=Tclk  UseAsADC=off  ADCChannel='1'  interface=AXI4-Lite  automatic_assignment=off  address_offset=hex2dec('90c')  intf_name=''  intf_description=''  timing_constraint=None  locs_specified=off  LOCs={}  io_standard={}  inherit_from_input=off  hdl_port=on  dbl_ovrd=off  block_type=gatewayin
  toDsp_config104 : xbsIndex_r4/Gateway In  gui_display_data_type=Fixed-point  arith_type=Unsigned  n_bits=32  bin_pt=0  preci_type=Single  exp_width=8  frac_width=24  rows=1  columns=1  quantization=Truncate  overflow=Wrap  period=Tclk  UseAsADC=off  ADCChannel='1'  interface=AXI4-Lite  automatic_assignment=off  address_offset=hex2dec('910')  intf_name=''  intf_description=''  timing_constraint=None  locs_specified=off  LOCs={}  io_standard={}  inherit_from_input=off  hdl_port=on  dbl_ovrd=off  block_type=gatewayin
  toDsp_config105 : xbsIndex_r4/Gateway In  gui_display_data_type=Fixed-point  arith_type=Unsigned  n_bits=32  bin_pt=0  preci_type=Single  exp_width=8  frac_width=24  rows=1  columns=1  quantization=Truncate  overflow=Wrap  period=Tclk  UseAsADC=off  ADCChannel='1'  interface=AXI4-Lite  automatic_assignment=off  address_offset=hex2dec('914')  intf_name=''  intf_description=''  timing_constraint=None  locs_specified=off  LOCs={}  io_standard={}  inherit_from_input=off  hdl_port=on  dbl_ovrd=off  block_type=gatewayin
  toDsp_config106 : xbsIndex_r4/Gateway In  gui_display_data_type=Fixed-point  arith_type=Unsigned  n_bits=32  bin_pt=0  preci_type=Single  exp_width=8  frac_width=24  rows=1  columns=1  quantization=Truncate  overflow=Wrap  period=Tclk  UseAsADC=off  ADCChannel='1'  interface=AXI4-Lite  automatic_assignment=off  address_offset=hex2dec('918')  intf_name=''  intf_description=''  timing_constraint=None  locs_specified=off  LOCs={}  io_standard={}  inherit_from_input=off  hdl_port=on  dbl_ovrd=off  block_type=gatewayin
  toDsp_config107 : xbsIndex_r4/Gateway In  gui_display_data_type=Fixed-point  arith_type=Unsigned  n_bits=32  bin_pt=0  preci_type=Single  exp_width=8  frac_width=24  rows=1  columns=1  quantization=Truncate  overflow=Wrap  period=Tclk  UseAsADC=off  ADCChannel='1'  interface=AXI4-Lite  automatic_assignment=off  address_offset=hex2dec('91c')  intf_name=''  intf_description=''  timing_constraint=None  locs_specified=off  LOCs={}  io_standard={}  inherit_from_input=off  hdl_port=on  dbl_ovrd=off  block_type=gatewayin
  toDsp_config108 : xbsIndex_r4/Gateway In  gui_display_data_type=Fixed-point  arith_type=Unsigned  n_bits=32  bin_pt=0  preci_type=Single  exp_width=8  frac_width=24  rows=1  columns=1  quantization=Truncate  overflow=Wrap  period=Tclk  UseAsADC=off  ADCChannel='1'  interface=AXI4-Lite  automatic_assignment=off  address_offset=hex2dec('920')  intf_name=''  intf_description=''  timing_constraint=None  locs_specified=off  LOCs={}  io_standard={}  inherit_from_input=off  hdl_port=on  dbl_ovrd=off  block_type=gatewayin
  toDsp_config109 : xbsIndex_r4/Gateway In  gui_display_data_type=Fixed-point  arith_type=Unsigned  n_bits=32  bin_pt=0  preci_type=Single  exp_width=8  frac_width=24  rows=1  columns=1  quantization=Truncate  overflow=Wrap  period=Tclk  UseAsADC=off  ADCChannel='1'  interface=AXI4-Lite  automatic_assignment=off  address_offset=hex2dec('924')  intf_name=''  intf_description=''  timing_constraint=None  locs_specified=off  LOCs={}  io_standard={}  inherit_from_input=off  hdl_port=on  dbl_ovrd=off  block_type=gatewayin
  toDsp_config110 : xbsIndex_r4/Gateway In  gui_display_data_type=Fixed-point  arith_type=Unsigned  n_bits=32  bin_pt=0  preci_type=Single  exp_width=8  frac_width=24  rows=1  columns=1  quantization=Truncate  overflow=Wrap  period=Tclk  UseAsADC=off  ADCChannel='1'  interface=AXI4-Lite  automatic_assignment=off  address_offset=hex2dec('928')  intf_name=''  intf_description=''  timing_constraint=None  locs_specified=off  LOCs={}  io_standard={}  inherit_from_input=off  hdl_port=on  dbl_ovrd=off  block_type=gatewayin
  toDsp_config111 : xbsIndex_r4/Gateway In  gui_display_data_type=Fixed-point  arith_type=Unsigned  n_bits=32  bin_pt=0  preci_type=Single  exp_width=8  frac_width=24  rows=1  columns=1  quantization=Truncate  overflow=Wrap  period=Tclk  UseAsADC=off  ADCChannel='1'  interface=AXI4-Lite  automatic_assignment=off  address_offset=hex2dec('92c')  intf_name=''  intf_description=''  timing_constraint=None  locs_specified=off  LOCs={}  io_standard={}  inherit_from_input=off  hdl_port=on  dbl_ovrd=off  block_type=gatewayin
  toDsp_config2 : xbsIndex_r4/Gateway In  gui_display_data_type=Fixed-point  arith_type=Unsigned  n_bits=32  bin_pt=12  preci_type=Single  exp_width=8  frac_width=24  rows=1  columns=1  quantization=Truncate  overflow=Wrap  period=Tclk  UseAsADC=off  ADCChannel='1'  interface=AXI4-Lite  automatic_assignment=off  address_offset=hex2dec('808')  intf_name=''  intf_description=''  timing_constraint=None  locs_specified=off  LOCs={}  io_standard={}  inherit_from_input=off  hdl_port=on  dbl_ovrd=off  block_type=gatewayin
  toDsp_config3 : xbsIndex_r4/Gateway In  gui_display_data_type=Fixed-point  arith_type=Unsigned  n_bits=32  bin_pt=0  preci_type=Single  exp_width=8  frac_width=24  rows=1  columns=1  quantization=Truncate  overflow=Wrap  period=Tclk  UseAsADC=off  ADCChannel='1'  interface=AXI4-Lite  automatic_assignment=off  address_offset=hex2dec('80c')  intf_name=''  intf_description=''  timing_constraint=None  locs_specified=off  LOCs={}  io_standard={}  inherit_from_input=off  hdl_port=on  dbl_ovrd=off  block_type=gatewayin
  toDsp_config4 : xbsIndex_r4/Gateway In  gui_display_data_type=Fixed-point  arith_type=Unsigned  n_bits=32  bin_pt=0  preci_type=Single  exp_width=8  frac_width=24  rows=1  columns=1  quantization=Truncate  overflow=Wrap  period=Tclk  UseAsADC=off  ADCChannel='1'  interface=AXI4-Lite  automatic_assignment=off  address_offset=hex2dec('810')  intf_name=''  intf_description=''  timing_constraint=None  locs_specified=off  LOCs={}  io_standard={}  inherit_from_input=off  hdl_port=on  dbl_ovrd=off  block_type=gatewayin
  toDsp_config5 : xbsIndex_r4/Gateway In  gui_display_data_type=Fixed-point  arith_type=Unsigned  n_bits=32  bin_pt=0  preci_type=Single  exp_width=8  frac_width=24  rows=1  columns=1  quantization=Truncate  overflow=Wrap  period=Tclk  UseAsADC=off  ADCChannel='1'  interface=AXI4-Lite  automatic_assignment=off  address_offset=hex2dec('814')  intf_name=''  intf_description=''  timing_constraint=None  locs_specified=off  LOCs={}  io_standard={}  inherit_from_input=off  hdl_port=on  dbl_ovrd=off  block_type=gatewayin
  toDsp_config511 : xbsIndex_r4/Gateway In  gui_display_data_type=Fixed-point  arith_type=Unsigned  n_bits=32  bin_pt=0  preci_type=Single  exp_width=8  frac_width=24  rows=1  columns=1  quantization=Truncate  overflow=Wrap  period=Tclk  UseAsADC=off  ADCChannel='1'  interface=AXI4-Lite  automatic_assignment=off  address_offset=hex2dec('FFC')  intf_name=''  intf_description=''  timing_constraint=None  locs_specified=off  LOCs={}  io_standard={}  inherit_from_input=off  hdl_port=on  dbl_ovrd=off  block_type=gatewayin
  toDsp_config6 : xbsIndex_r4/Gateway In  gui_display_data_type=Fixed-point  arith_type=Unsigned  n_bits=32  bin_pt=0  preci_type=Single  exp_width=8  frac_width=24  rows=1  columns=1  quantization=Truncate  overflow=Wrap  period=Tclk  UseAsADC=off  ADCChannel='1'  interface=AXI4-Lite  automatic_assignment=off  address_offset=hex2dec('818')  intf_name=''  intf_description=''  timing_constraint=None  locs_specified=off  LOCs={}  io_standard={}  inherit_from_input=off  hdl_port=on  dbl_ovrd=off  block_type=gatewayin
  Out1 : Outport
  Out2 : Outport  Port=2
  Out3 : Outport  Port=3
  Out4 : Outport  Port=4
  Out5 : Outport  Port=5
  tag scope: Ampl0=global, Ampl1=global, BW=global, ConfigReg0=global, F0=global, F10=global, F11=global, F1=global, F2=global, F3=global, F4=global, F5=global, F6=global, F7=global, F8=global, F9=global, FBen=global, FBgain=global, FBlimit=global, FBreset=global, NotchSimEn=global, RFen=global, RefSource=global, dFsb=global, debugMux=global, fbPolarity=global, refDel=global, whiteNoiseGen=global
  wires:
  config0/1 -> toDsp_config0/1
  toDsp_config0/1 -> Register2/1
  fromDsp_status0/1 -> Ampl Mon/1, Out1/1
  config4/1 -> toDsp_config4/1
  toDsp_config4/1 -> Register3/1
  fromDsp_status1/1 -> Ampl Mon/2, Out2/1
  config5/1 -> toDsp_config5/1
  toDsp_config5/1 -> Register4/1
  fromDsp_status2/1 -> Ampl Mon/3, Out3/1
  "Fi 0 "/1 -> toDsp_config100/1
  toDsp_config100/1 -> Register5/1
  fromDsp_status3/1 -> Ampl Mon/4, Out4/1
  config63/1 -> toDsp_cmd0/1
  toDsp_cmd0/1 -> Register6/1
  Register3/1 -> Slice6/1, Slice5/1
  Register5/1 -> BitBasher1/1
  Register6/1 -> Slice4/1, Gateway Out1/1
  Slice5/1 -> Reinterpret/1
  Slice6/1 -> Reinterpret1/1
  Register4/1 -> BitBasher13/1, BitBasher12/1
  Register2/1 -> Gateway Out6/1, [ConfigReg0], Slice/1, Slice1/1, Slice2/1, Slice3/1, Slice7/1, Slice9/1
  Slice1/1 -> [RefSource]
  Slice/1 -> [RFen]
  Slice2/1 -> [NotchSimEn]
  Slice3/1 -> [whiteNoiseGen]
  Reinterpret/1 -> [Ampl0]
  Reinterpret1/1 -> [Ampl1]
  Gateway Out6/1 -> Control Reg/1
  Gateway Out/1 -> F0/1
  Slice4/1 -> [FBreset]
  BitBasher13/1 -> [dFsb]
  BitBasher12/1 -> [FBlimit]
  BitBasher1/1 -> Gateway Out/1, [F0]
  Gateway Out1/1 -> Out5/1
  [FBreset] -> Terminator3/1
  [NotchSimEn] -> Terminator2/1
  fromDsp_status7/1 -> Terminator9/1
  fromDsp_status6/1 -> Terminator8/1
  [F0] -> Convert/1, Slice10/1, fromDsp_status6/1
  fromDsp_status5/1 -> Ampl Mon/6, Terminator10/1
  Slice9/1 -> [debugMux]
  [F1] -> Slice11/1, Convert1/1, fromDsp_status7/1
  [F0] -> fromDsp_status4/1
  [F0] -> fromDsp_status1/1
  [F0] -> fromDsp_status3/1
  [F0] -> fromDsp_status2/1
  [F0] -> fromDsp_status0/1
  fromDsp_status4/1 -> Ampl Mon/5, Terminator4/1
  [F0] -> fromDsp_status5/1
  fromdsp_debug1_1/1 -> Terminator15/1
  fromdsp_debug1_0/1 -> Terminator14/1
  fromdsp_debug0_1/1 -> Terminator13/1
  fromdsp_debug0_0/1 -> Terminator12/1
  Slice10/1 -> Reinterpret7/1
  Convert/1 -> Reinterpret6/1
  Slice11/1 -> Reinterpret8/1
  Reinterpret9/1 -> fromdsp_debug1_0/1
  Reinterpret6/1 -> fromdsp_debug0_0/1
  Reinterpret7/1 -> fromdsp_debug0_1/1
  Convert1/1 -> Reinterpret9/1
  Reinterpret8/1 -> fromdsp_debug1_1/1
  In13/1 -> toDsp_config511/1
  toDsp_config511/1 -> Register11/1
  Register11/1 -> fromDsp_status511/1
  fromDsp_status511/1 -> Terminator16/1
  config1/1 -> toDsp_config1/1
  toDsp_config1/1 -> Register12/1
  config2/1 -> toDsp_config2/1
  toDsp_config2/1 -> Register13/1
  config3/1 -> toDsp_config3/1
  toDsp_config3/1 -> Register14/1
  Slice12/1 -> [FBen]
  Register12/1 -> Slice12/1
  BitBasher15/1 -> [FBgain]
  Register13/1 -> BitBasher15/1
  Slice14/1 -> [refDel]
  Register14/1 -> Slice14/1
  config6/1 -> toDsp_config6/1
  toDsp_config6/1 -> Register15/1
  Slice15/1 -> Reinterpret10/1
  Register15/1 -> Slice15/1
  Reinterpret10/1 -> [BW]
  Fi 1/1 -> toDsp_config101/1
  toDsp_config101/1 -> Register16/1
  Register16/1 -> BitBasher2/1
  Gateway Out2/1 -> F1/1
  BitBasher2/1 -> Gateway Out2/1, [F1]
  Fi 2/1 -> toDsp_config102/1
  toDsp_config102/1 -> Register18/1
  Register18/1 -> BitBasher3/1
  Gateway Out3/1 -> F2/1
  BitBasher3/1 -> Gateway Out3/1, [F2]
  Fi 3/1 -> toDsp_config103/1
  toDsp_config103/1 -> Register17/1
  Register17/1 -> BitBasher4/1
  Gateway Out4/1 -> F3/1
  BitBasher4/1 -> Gateway Out4/1, [F3]
  Fi 4/1 -> toDsp_config104/1
  toDsp_config104/1 -> Register22/1
  Register22/1 -> BitBasher5/1
  Gateway Out5/1 -> F4/1
  BitBasher5/1 -> Gateway Out5/1, [F4]
  Fi 5/1 -> toDsp_config105/1
  toDsp_config105/1 -> Register19/1
  Register19/1 -> BitBasher6/1
  Gateway Out7/1 -> F5/1
  BitBasher6/1 -> Gateway Out7/1, [F5]
  Fi 6/1 -> toDsp_config106/1
  toDsp_config106/1 -> Register21/1
  Register21/1 -> BitBasher7/1
  Gateway Out8/1 -> F6/1
  BitBasher7/1 -> Gateway Out8/1, [F6]
  Fi 7/1 -> toDsp_config107/1
  toDsp_config107/1 -> Register20/1
  Register20/1 -> BitBasher8/1
  Gateway Out9/1 -> F7/1
  BitBasher8/1 -> Gateway Out9/1, [F7]
  Fi 8/1 -> toDsp_config108/1
  toDsp_config108/1 -> Register26/1
  Register26/1 -> BitBasher9/1
  Gateway Out10/1 -> F8/1
  BitBasher9/1 -> Gateway Out10/1, [F8]
  Fi 9/1 -> toDsp_config109/1
  toDsp_config109/1 -> Register23/1
  Register23/1 -> BitBasher10/1
  Gateway Out11/1 -> F9/1
  BitBasher10/1 -> Gateway Out11/1, [F9]
  Fi 10/1 -> toDsp_config110/1
  toDsp_config110/1 -> Register25/1
  Register25/1 -> BitBasher11/1
  Gateway Out12/1 -> F10/1
  BitBasher11/1 -> Gateway Out12/1, [F10]
  Fi 11/1 -> toDsp_config111/1
  toDsp_config111/1 -> Register24/1
  Register24/1 -> BitBasher14/1
  Gateway Out13/1 -> F11/1
  BitBasher14/1 -> Gateway Out13/1, [F11]
  Slice7/1 -> [fbPolarity]
  [RefSource] -> Terminator1/1

== system CryoDetFP/DspCore/DAC demux clock ==
  note: Use DAC clock to generate edge to synchronize simulation of DAC demuxing in FPGA VHDL wrapper
      | output 1 = I
      | 0 = Q
      | This generates no code in FPGA, it is just  here to make Simulink simulation run
  In1 : Inport
  Add : Sum
  Clock Enable Probe : xbsIndex_r4/Clock Enable Probe  inherit_constraints=on  block_type=ceprobe
      settings: infoedit="Clock enable extractor.  Produces a Boolean output that mirrors the hardware clock enable associated with the input sample rate.<br><br>Hardware notes: in hardware this block costs nothing."
  Constant : Constant  Value=2
  Down Sample : xbsIndex_r4/Down Sample  sample_ratio=2  sample_phase="Last Value of Frame  (most efficient)"  en=off  rst=off  latency=1  dbl_ovrd=off  block_type=dsamp
  Math Function : Math  Operator=mod  SaturateOnIntegerOverflow=on
  Transport Delay : TransportDelay  DelayTime=Tclk/2
  fromdsp_dacdata1_2 : xbsIndex_r4/Gateway Out  inherit_from_input=off  hdl_port=off  rows=1  columns=1  UseAsDAC=off  DACChannel='1'  interface=None  automatic_assignment=on  address_offset=hex2dec('00')  intf_name=''  intf_description=''  timing_constraint=None  locs_specified=off  LOCs={}  io_standard={}  block_type=gatewayout
  IQtoggle : Outport
  wires:
  Clock Enable Probe/1 -> fromdsp_dacdata1_2/1
  Down Sample/1 -> Clock Enable Probe/1
  In1/1 -> Down Sample/1
  fromdsp_dacdata1_2/1 -> Add/1, Transport Delay/1
  Transport Delay/1 -> Add/2
  Add/1 -> Math Function/1
  Math Function/1 -> IQtoggle/1
  Constant/1 -> Math Function/2
